simulink model "Sim4Tanks"  (R2021b)
settings: Solver=FixedStepAuto  StartTime=0.0  StopTime=Tf  FixedStep=Ts  RelTol=1e-3
settings Model: Creator=Mohamed Yagoubi  LastModifiedBy=Mohamed Yagoubi

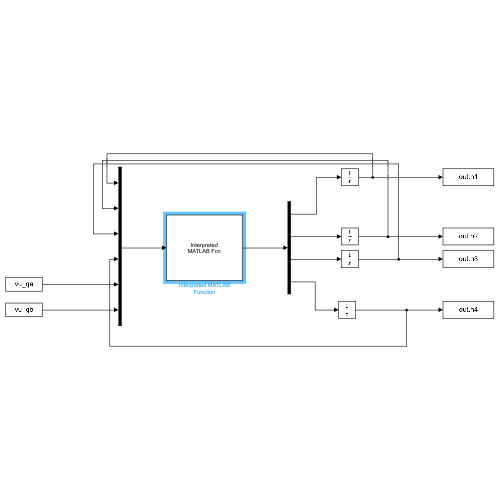
[thumbnail: Simulink's stored preview of the top-level diagram]
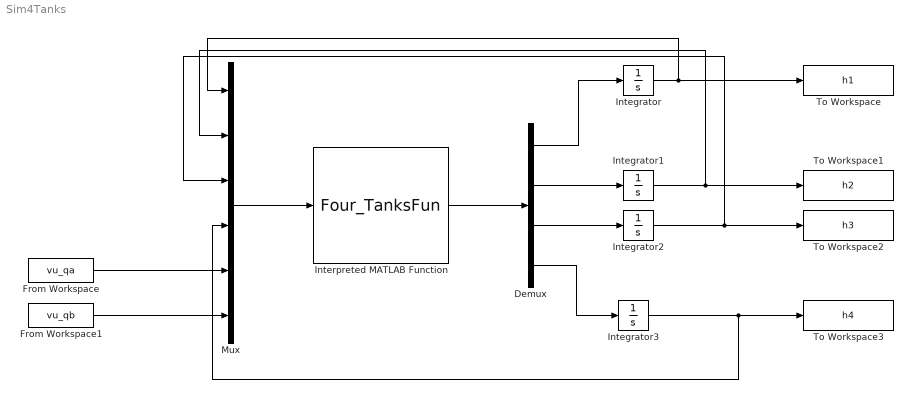
== system Sim4Tanks ==
  Demux : Demux
  From Workspace : FromWorkspace  VariableName=vu_qa
  From Workspace1 : FromWorkspace  VariableName=vu_qb
  Integrator{,1..3} (4 alike) : Integrator
  Interpreted MATLAB Function : MATLABFcn  MATLABFcn=Four_TanksFun  OutputDimensions=4
  Mux : Mux  Inputs=6
  To Workspace : ToWorkspace  VariableName=h1  SaveFormat=Timeseries  SampleTime=-1
  To Workspace1 : ToWorkspace  VariableName=h2  SaveFormat=Timeseries  SampleTime=-1
  To Workspace2 : ToWorkspace  VariableName=h3  SaveFormat=Timeseries  SampleTime=-1
  To Workspace3 : ToWorkspace  VariableName=h4  SaveFormat=Timeseries  SampleTime=-1
  wires:
  Mux/1 -> Interpreted MATLAB Function/1
  Interpreted MATLAB Function/1 -> Demux/1
  Demux/1 -> Integrator/1
  Demux/2 -> Integrator1/1
  Demux/3 -> Integrator2/1
  Demux/4 -> Integrator3/1
  Integrator/1 -> To Workspace/1, Mux/1
  Integrator1/1 -> To Workspace1/1, Mux/2
  Integrator2/1 -> To Workspace2/1, Mux/3
  Integrator3/1 -> To Workspace3/1, Mux/4
  From Workspace/1 -> Mux/5
  From Workspace1/1 -> Mux/6
